simulink model "Planta_com_Controle"  (Simulink 8.7)
settings: Solver=VariableStepAuto  StartTime=0.0  StopTime=inf  RelTol=1e-3
settings Model: Creator=Tiago  LastModifiedBy=Tiago
settings DataIOCC: LimitDataPoints=off  SaveFormat=Dataset
settings DebuggingCC: UnderspecifiedInitializationDetection=Simplified  MergeDetectMultiDrivingBlocksExec=error
settings HardwareCC: ProdBitPerPointer=64  ProdLargestAtomicFloat=Float  ProdIntDivRoundTo=Zero  ProdEndianess=LittleEndian  ProdWordSize=64  ProdHWDeviceType=Intel->x86-64 (Windows64)
settings ModelReferenceCC: PropagateSignalLabelsOutOfModel=on
settings ConfigComp: CovModelRefEnable=off

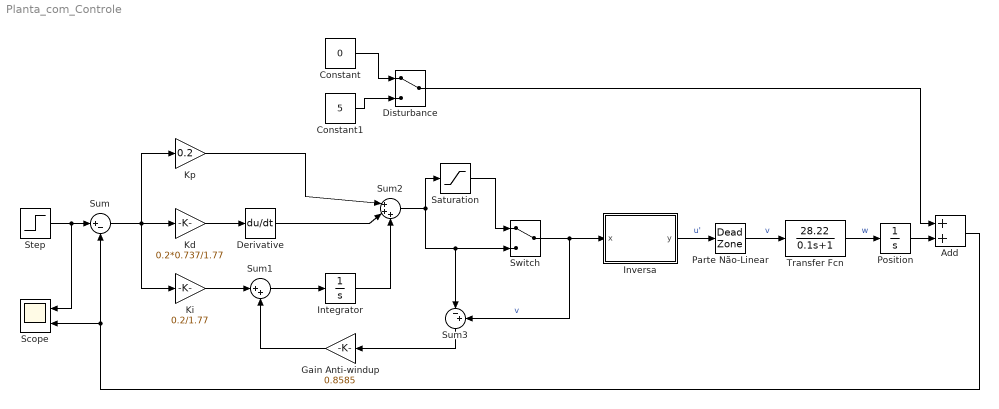
== system Planta_com_Controle ==
  Add : Sum
  Constant : Constant  Value=0
  Constant1 : Constant  Value=5
  Derivative : Derivative
  Disturbance : ManualSwitch
  Gain Anti-windup : Gain  Gain=0.8585
  Integrator : Integrator
  Inversa : MATLAB Function  TreatAsAtomicUnit=on
  Kd : Gain  Gain=0.2*0.737/1.77
  Ki : Gain  Gain=0.2/1.77
  Kp : Gain  Gain=0.2
  Parte Não-Linear : DeadZone  LowerValue=-0.5296  UpperValue=0.5635  SaturateOnIntegerOverflow=on
  Position : Integrator
  Saturation : Saturate  UpperLimit=2  LowerLimit=-2
  Scope : Scope  NumInputPorts=2
  Step : Step  SampleTime=0
  Sum : Sum  Inputs=|+-
  Sum1 : Sum  Inputs=|++
  Sum2 : Sum  Inputs=|+++
  Sum3 : Sum  Inputs=|-+
  Switch : ManualSwitch
  Transfer Fcn : TransferFcn  Numerator=[28.22]  Denominator=[0.1 1]
  wires:
  Parte Não-Linear/1 -> Transfer Fcn/1  "v"
  Add/1 -> Scope/2, Sum/2
  Kd/1 -> Derivative/1
  Kp/1 -> Sum2/1
  Derivative/1 -> Sum2/2
  Integrator/1 -> Sum2/3
  Sum3/1 -> Gain Anti-windup/1
  Saturation/1 -> Switch/1
  Sum2/1 -> Sum3/1, Switch/2, Saturation/1
  Inversa/1(y) -> Parte Não-Linear/1  "u'"
  Ki/1 -> Sum1/1
  Sum1/1 -> Integrator/1
  Transfer Fcn/1 -> Position/1  "w"
  Step/1 -> Scope/1, Sum/1
  Switch/1 -> Sum3/2, Inversa/1(x)  "v"
  Sum/1 -> Kp/1, Ki/1, Kd/1
  Position/1 -> Add/2
  Disturbance/1 -> Add/1
  Constant/1 -> Disturbance/1
  Constant1/1 -> Disturbance/2
  Gain Anti-windup/1 -> Sum1/2

== matlab function Inversa ==
  data: x input double; y output double
function y = fcn(x)
    if(x >= 0.5635)
        x = x + 0.5635;
    elseif(x > -0.5296 && x < 0.5635) 
        x = 0;
    end
    if(x <= -0.5296)
        x = x - 0.5296;
    end
y = x;
